simulink library "base_lib"  (R2023a)
settings: Solver=VariableStepAuto  StartTime=0.0  StopTime=10.0  RelTol=1e-3
(part 3 of 4)

== matlab function base_lib/F0010_gasFlow/F0010_mixtureProperties.m ==
  data: p input; x output; cp_m output; cv_m output; R_m output; par parameter
function [x, cp_m, cv_m, R_m] = F0010_mixtureProperties(p, par)
% Parameters
cp_j = par.cp_j; % [J/kgK]  - Specific heats
M_j  = par.M_j;  % [kg/mol] - Molar masses
R_j  = par.R_j;  % [J/kgK]  - Specific gas constant

% Mole fractions
p_tot = sum(p);
x     = p ./ p_tot;

% Average molar mass
M_avg = sum(x .* M_j);

% Mole fraction to mass fraction
w = x .* M_j ./ M_avg;

% Mixture gas constant
R_m = sum(w .* R_j);

% Mixture specific heats
cp_m = sum(w .* cp_j);
cv_m = cp_m - R_m;

end

== matlab function base_lib/F0001_panasonicCell/F0001_ocvSOC.m ==
  data: SOC input; U output
% A Generalized SOC-OCV Model for Lithium-Ion
% Batteries and the SOC Estimation for LNMCO Battery
% Zhang et al, Energies
% doi:10.3390/en9110900

% Fit to OCV-data from
% Li-Ion Battery Model Performance for Automotive Drive
% Cycles with Current Pulse and EIS Parameterization
% Kolmeyer et al, 
% 978-1-5090-3953-1/$31.00 ©2017 IEEE

function U = F0001_ocvSOC(SOC)
% inputs x [-] - state of charge

% parameters
a =  2.0966;
b = -0.0055;
c = -0.2433;
d =  2.3054;
m =  3.0965;
n =  0.6010;

% OCV
x = SOC;
U = a + b * (-log(x)).^m + c .* x + d.*exp( n.*(x-1));
end

== matlab function base_lib/F0010_gasFlow/F0010_multicomponentFlow.m ==
  data: p_us input; W_split output; W_tot input; par parameter
function W_split = F0010_multicomponentFlow(p_us, W_tot, par)
% Parameters
cp_j = par.cp_j; % [J/kgK]  - Specific heats
M_j  = par.M_j;  % [kg/mol] - Molar masses
R_j  = par.R_j;  % [J/kgK]  - Specific gas constant

% Mole fractions
p_tot = sum(p_us);
x     = p_us ./ p_tot;

% Average molar mass
M_avg = sum(x .* M_j);

% Mole fraction to mass fraction
w = x .* M_j ./ M_avg;

% outlet species convective mass flow
W_split = W_tot .* w;

end

== matlab function base_lib/F0010_gasFlow/F0010_pressureSupply.m ==
  data: p_tot input; p_out output; x_H2_dry input; x_O2_dry input; RH input; p_sat input; par parameter
function p_out = F0010_pressureSupply(p_tot, x_H2_dry, x_O2_dry, RH, p_sat, par)

% mole fraction of vapor
x_H2O = RH .* p_sat ./ p_tot;

% mole fraction hydrogen
x_H2 = (1-x_H2O).*x_H2_dry;

% mole fraction hydrogen
x_O2 = (1-x_H2O).*x_O2_dry;

% mole fraction nitrogen
x_N2 = 1 - x_H2 - x_O2 - x_H2O;




% partial pressures
p_out = [x_H2; x_O2; x_H2O; x_N2] .* p_tot;

end

== matlab function base_lib/F0010_gasFlow/F0010_pressureSupply2.m ==
  data: p_tot input; p_H2 output; x_H2_dry input; x_O2_dry input; RH input; p_sat input; p_O2 output; p_H2O output; p_N2 output; par parameter
function [p_H2, p_O2, p_H2O, p_N2] = F0010_pressureSupply2(p_tot, x_H2_dry, x_O2_dry, RH, p_sat, par)

% mole fraction of vapor
x_H2O = RH .* p_sat ./ p_tot;

% mole fraction hydrogen
x_H2 = (1-x_H2O).*x_H2_dry;

% mole fraction hydrogen
x_O2 = (1-x_H2O).*x_O2_dry;

% mole fraction nitrogen
x_N2 = 1 - x_H2 - x_O2 - x_H2O;

% output
p_H2  = x_H2  .* p_tot;
p_O2  = x_O2  .* p_tot;
p_H2O = x_H2O .* p_tot;
p_N2  = x_N2  .* p_tot;

end

== matlab function base_lib/F0010_gasFlow/F0010_pressureToMass.m ==
  data: p input; m output; T input; par parameter
function m = F0010_pressureToMass(p, T, par)
% parameters
Rj     = par.R_j;
V      = par.V;

% mass
m = p .* V ./ (Rj .* T);
end

== matlab function base_lib/F0010_gasFlow/F0010_throttleArea.m ==
  data: alpha input; A_t output; par parameter
function A_t = F0010_throttleArea(alpha, par)
% model parameters
a0 = par.a0;
a1 = par.a1;
a2 = par.a2;

% effective area
A_t = a0 + a1.*alpha + a2 .* alpha.^2;
end

== matlab function base_lib/F0011_ellipseCompressor/F0011_A.m ==
  data: N_corr_n input; A output; par parameter
function A = F0011_A(N_corr_n, par)
% parameters
u1 = N_corr_n;
u2 = par.C_a(1);
u3 = par.C_a(2);
u4 = par.C_a(3);
u5 = par.Delta_h_max;
u6 = par.Wc_max_map;

% output
A = -( u5./u6 ).*( u2.*u1 ./( (1 + u3.*u1.^2).^u4 ));
end

== matlab function base_lib/F0011_ellipseCompressor/F0011_B.m ==
  data: N_corr_n input; B output; par parameter
function B = F0011_B(N_corr_n, par)
% parameters
u1 = N_corr_n;
u2 = par.C_b(1);
u3 = par.C_b(2);
u4 = par.Delta_h_max;

% output
B = u4 .* ( u2 .* u1.^2 + u3 .* u1.^3 );
end

== matlab function base_lib/F0011_ellipseCompressor/F0011_CUR.m ==
  data: N_corr_n input; CUR output; par parameter
function CUR = F0011_CUR(N_corr_n, par)
% parameters
a1     = par.C_cur(1);
a2     = par.C_cur(2);
a3     = par.C_cur(3);

% Speed ratio
N = N_corr_n;

% output
CUR = a1 + a2.*N.^a3;
end

== matlab function base_lib/F0003_pukrushpan2004/F0003_diffusiveFlow.m ==
  data: lambda_an input; W output; lambda_m input; lambda_ca input; T input; par parameter
function W = F0003_diffusiveFlow(lambda_an, lambda_m, lambda_ca, T, par)

% parameters
A   = par.A_fc; % [cm2] - cell area
t_m = par.t_m;  % [cm]  - membrane thickness

% constants
F     = 96485;  % [C/mol]   - Faradays constant
R     = 8.314;  % [J/(molK] - gas constant 
M_H2O = 0.018;  % [kg/mol]  - water molecular mass

rho_mb_dry = 0.002; % [kg/cm^3] - membrane dry density;
M_mb_dry   = 1.1;   % [kg/mol]  - membrane dry equivalent weight 

% membrane diffusivity
D                  = 1e-6;
D(lambda_m >= 2)   = 1e-6 * (1 + 2*(lambda_m-2));
D(lambda_m >= 3)   = 1e-6 * (3 - 1.67*(lambda_m-3));
D(lambda_m >= 4.5) = 1.25e-6;
D_w                = 12 * D.*exp(2416*(1/303 - 1/T));

% Water concentrations on each side
c_an = rho_mb_dry ./ M_mb_dry .* lambda_an; % [mol/cm3] - water concentration at anode
c_ca = rho_mb_dry ./ M_mb_dry .* lambda_ca; % [mol/cm3] - water concentration at cathode

% Diffusive flow
W = M_H2O .* A .* D_w .* (c_an - c_ca)/t_m;

end

== matlab function base_lib/F0011_ellipseCompressor/F0011_K_loss.m ==
  data: W_corr input; K_loss output; N_corr input; par parameter
function K_loss = F0011_K_loss(W_corr, N_corr, par)
% parameters
rho1   = par.rho1;
D      = par.D_2;
C_loss = par.C_loss;

% output
K_loss = 1 + C_loss .* ( rho1.*D.^3 .* pi/60 ) .* (N_corr./W_corr);
end

== matlab function base_lib/F0011_ellipseCompressor/F0011_PI_ZSL.m ==
  data: N_corr_n input; PI_ZSL output; par parameter
function PI_ZSL = F0011_PI_ZSL(N_corr_n, par)
% parameters
PI_max = par.PI_max_map;
a1     = par.C_PIzs(1);
a2     = par.C_PIzs(2);

% Speed ratio
N = N_corr_n;

% output
PI_ZSL  = 1 + (PI_max - 1) .* ( a1.*N.^a2 );
end

== matlab function base_lib/F0011_ellipseCompressor/F0011_P_c.m ==
  data: W_c input; P_c output; T_us input; T_ds input; par parameter
function P_c = F0011_P_c(W_c, T_us, T_ds, par)
% parameters
cp  = par.Cp_air;

% compressor work
P_c = cp .* W_c .* (T_ds - T_us);
end

== matlab function base_lib/F0011_ellipseCompressor/F0011_Pi_ch.m ==
  data: N_corr_n input; Pi_ch output; par parameter
function Pi_ch = F0011_Pi_ch(N_corr_n, par)
% parameters
PI_max = par.PI_max_map;
a1     = par.C_PIch(1);
a2     = par.C_PIch(2);
a3     = par.C_PIch(3);

% Speed ratio
N = N_corr_n;

% output
Pi_ch  = PI_max .* ( a1 + a2.*N.^a3 );
end

== matlab function base_lib/F0011_ellipseCompressor/F0011_T_ds.m ==
  data: Pi_c input; T_ds output; T_us input; eta_c input; par parameter
function T_ds = F0011_T_ds(Pi_c, T_us, eta_c, par)
% model constants
g = par.gamma_air;

% compressor out temperature (adiabatic)
T_ds = T_us + T_us ./ eta_c .* ( Pi_c.^((g-1)/g)  - 1  );
end

== matlab function base_lib/F0011_ellipseCompressor/F0011_W_ZSL.m ==
  data: N_corr_n input; W_ZSL output; par parameter
function W_ZSL = F0011_W_ZSL(N_corr_n, par)
% parameters
Wc_max = par.Wc_max_map;
a1     = par.C_Wzs(1);
a2     = par.C_Wzs(2);

% Speed ratio
N = N_corr_n;

% output
W_ZSL = Wc_max .* a1 .* N.^a2;
end

== matlab function base_lib/F0011_ellipseCompressor/F0011_W_ch_atan.m ==
  data: N_corr_n input; W_ch_atan output; par parameter
function W_ch_atan = F0011_W_ch_atan(N_corr_n, par)
% parameters
Wc_max = par.Wc_max_map;
a1     = par.C_Wch(1);
a2     = par.C_Wch(2);
a3     = par.C_Wch(3);
a4     = par.C_Wch(4);

% Speed ratio
N = N_corr_n;

% output
W_ch_atan = Wc_max .* (a1 + a2 .* atan( a3.*N - a4));
end

== matlab function base_lib/F0011_ellipseCompressor/F0011_dTq.m ==
  data: Tq_em input; dw_c output; Tq_c input; w_c input; par parameter
function dw_c = F0011_dTq(Tq_em, Tq_c, w_c, par)
% parameters
J_c = par.J_c;
c   = par.c_fric;

% shaft friction
Mf = c .* w_c;

% turbo shaft dynamics
% Model 8.3
dw_c = 1/J_c .* ( Tq_em - Tq_c - Mf);

end

== matlab function base_lib/F0011_ellipseCompressor/F0011_dh_act.m ==
  data: W_c_corr input; dh_act output; K_loss input; B input; A input
function dh_act = F0011_dh_act(W_c_corr, K_loss, B, A)
% inputs
u1 = W_c_corr;
u2 = K_loss;
u3 = B;
u4 = A;

% actual enthalpy change
dh_act = u2 .* ( u3 + u4 .* u1 );

end

== matlab function base_lib/F0011_ellipseCompressor/F0011_dh_is.m ==
  data: Pi_c input; dh_is output; par parameter
function dh_is = F0011_dh_is(Pi_c, par)
% inputs
u1 = Pi_c;

% parameters
cp_air = par.Cp_air;
T_ref  = par.T_ref;
g      = par.gamma_air;

% isentropic enthalpy change
dh_is = cp_air .* T_ref .* ( u1.^((g - 1)./g) - 1 );
end

== matlab function base_lib/F0011_ellipseCompressor/F0011_ellipseModel.m ==
  data: Pi_c input; W_corr output; Pi_ch input; PI_ZSL input; CUR input; W_ZSL input; W_ch input; par parameter
function W_corr = F0011_ellipseModel(Pi_c, Pi_ch, PI_ZSL, CUR, W_ZSL, W_ch, par)
% inputs
u1 = min(Pi_c, PI_ZSL);
u2 = Pi_ch;
u3 = PI_ZSL;
u4 = CUR;
u5 = W_ZSL;
u6 = W_ch;


% inputs
u1 = min(Pi_c, PI_ZSL);
u2 = Pi_ch;
u3 = PI_ZSL;
u4 = CUR;
u5 = W_ZSL;
u6 = W_ch;

% Surge / Regular / Choke
if (Pi_c >  PI_ZSL)
    W_corr = W_ZSL - (Pi_c - PI_ZSL)./par.alpha_kPiW0;
elseif (Pi_c < Pi_ch)
    W_corr = W_ch;
else
    W_corr = u5 + (u6-u5).*( (1 - ( (u1-u2)./(u3-u2) ).^u4).^(1./u4) );
end

== matlab function base_lib/F0011_ellipseCompressor/F0011_ellipseModelPressure.m ==
  data: W_corr input; Pi_c output; Pi_ch input; PI_ZSL input; CUR input; W_ZSL input; W_ch input; par parameter
function Pi_c = F0011_ellipseModelPressure(W_corr, Pi_ch, PI_ZSL, CUR, W_ZSL, W_ch, par)

% inputs
W_corr = min(W_corr, W_ch);
W_corr = max(W_corr, W_ZSL);

% Surge / Regular / Choke
if (W_corr <  W_ZSL)
    Pi_c = PI_ZSL;
elseif (W_corr > W_ch)
    Pi_c = Pi_ch;
else
    Pi_c   = Pi_ch + ...
    (PI_ZSL - Pi_ch) .* ... 
    (1 - ((W_corr - W_ZSL)./(W_ch - W_ZSL)).^CUR ).^(1./CUR);
end

== matlab function base_lib/F0003_pukrushpan2004/F0003_dragFlow.m ==
  data: I input; W output; lambda input
function W = F0003_dragFlow(I, lambda)

% parameters
F          = 96485;  % [C/mol]   - Faradays constant
M_H2O      = 0.018;  % [kg/mol]  - water molecular mass

% electro-osmotic drag coefficient
n_d = 0.0029 .* lambda.^2 + 0.05 .* lambda;

% Drag flow
W =  M_H2O .* n_d .* I / F;
end

== matlab function base_lib/F0011_ellipseCompressor/F0011_flowCorrection.m ==
  data: W_c input; W_corr output; p1 input; T1 input; par parameter
function W_corr = F0011_flowCorrection(W_c, p1, T1,  par)

% corrected flow
W_corr = W_c .* sqrt( T1./par.T_ref) ./ (p1./par.p_ref);

end

== matlab function base_lib/F0011_ellipseCompressor/F0011_linearSurgeFlow.m ==
  data: W_ZSL input; W_corr_surge output; Pi_ZSL input; Pi_c input; par parameter
function W_corr_surge = F0011_linearSurgeFlow(W_ZSL, Pi_ZSL, Pi_c, par)
% Surge flow
W_corr_surge = W_ZSL - (Pi_c - Pi_ZSL)./par.alpha_kPiW0;

% Saturation
W_corr_surge(W_corr_surge < 1e-4) = 1e-4;
end

== matlab function base_lib/F0014_titanXradiator/F0014_condenserPressureDrop.m ==
  data: T input; dp output; p input; W input; par parameter
function dp = F0014_condenserPressureDrop(T, p, W, par)

% parameters
StS  = par.StS;
HtH  = par.HtH;
R    = par.R_air;
c_dp = par.c_dp; 

% Area
A = StS .* HtH;

% Velocity
v = W .* R .* T ./ (p.*A);

% pressure drop
dp = c_dp(1) .* v.^2 + c_dp(2) .* v;

== matlab function base_lib/F0014_titanXradiator/F0014_coreFlowDelay.m ==
  data: W input; t output; rho input; par parameter
function t = F0014_coreFlowDelay(W, rho, par)

% parameters
HtH = par.HtH;
StS = par.StS;
CdT = par.CdT;

% approximate core inner flow area
A = 0.15 .* CdT .* StS;

% flow velocity
v = max(W ./ ( rho .* A), 0.01);

% time delay
t = min(HtH ./ v, 20);

== matlab function base_lib/F0014_titanXradiator/F0014_epsCrossFlowUnmixed.m ==
  data: NTU input; e output; C input
function e = F0014_epsCrossFlowUnmixed(NTU, C)
N = NTU;
% N = max(N, 0);
n = N.^(-0.22);

% tanhyp switch for C approaching zero
y = (tanh(C*1e2 - pi) + 1 )./2;

% Holman, Table 10.3, Cross flow, both fluids unmixed:
e1  = 1 - exp( ( exp( -N.*C.*n ) - 1 )./(C.*n) );

% C = 0
e0 = 1 - exp(-N);

% output
e = y.*e1 + (1-y).*e0;

== matlab function base_lib/F0014_titanXradiator/F0014_fanAffinityLaw.m ==
  data: n1 input; q1 output; q2 input; dp1 output; P1 output; par parameter
function [q1, dp1, P1] = F0014_fanAffinityLaw(n1, q2, par)
% Source:
% https://www.engineeringtoolbox.com/fan-affinity-laws-d_196.html

% parameters
dp2 = par.dp2;
P2  = par.P2;
n2  = par.n2;
d1  = par.d1;
d2  = par.d2;

% Affinity laws
q1  = q2  .* (n1./n2)    .* (d1./d2).^3;
dp1 = dp2 .* (n1./n2).^2 .* (d1./d2).^2;
P1  = P2  .* (n1./n2).^3 .* (d1./d2).^5;

== matlab function base_lib/F0014_titanXradiator/F0014_fanCurve.m ==
  data: q input; dp output; dp0_n input; par parameter
function dp = F0014_fanCurve(q, dp0_n, par)

% parameters
dpr = par.dpr;
dp0 = par.dp0;
q0  = par.q0;

% pressure drop/increase
temp = (q ./ q0).^2;
dp   = max(dpr .* temp, dp0_n - dp0 .* temp);

== matlab function base_lib/F0014_titanXradiator/F0014_heatCapacityRates.m ==
  data: W_air input; C_min output; W_cl input; cp_cl input; C_max output; C_air output; C_cl output; par parameter
function [C_min, C_max, C_air, C_cl] = F0014_heatCapacityRates(W_air, W_cl, cp_cl, par)

% parameters
cp_air = par.cp_air;
% cp_clt = par.cp_clt;

% heat capacity rates
C_air = W_air.*cp_air;
C_cl = W_cl.*cp_cl;

% max/min rates
C_min = min(C_air, C_cl);
C_max = max(C_air, C_cl);

== matlab function base_lib/F0003_pukrushpan2004/F0003_outputVoltage.m ==
  data: I input; V output; p_an input; p_ca input; p_sat input; lambda_m input; T input; Q_gen output; par parameter
function [V, Q_gen] = F0003_outputVoltage(I, p_an, p_ca, p_sat, lambda_m, T, par)
% ref: Control-Oriented Modeling and Analysis for Automotive Fuel Cell Systems
% authors: Jay T. Pukrushpan, Huei Peng, Anna G. Stefanopoulou
% J. Dyn. Sys., Meas., Control. Mar 2004
% https://doi.org/10.1115/1.1648308

% specify output sizes
Q_gen = 0;
V     = 0;

% parameters
A = par.A_fc; % [cm2]       - cell area
j = I ./ A;

% partial pressures
p_H2     = p_an(1); % [Pa] - hydrogen partial pressure
% p_H2O_an = p_an(2); % [Pa] - water --
% p_N2_an  = p_an(3); % [Pa] - nitrogen --
p_O2     = p_ca(2); % [Pa] - oxygen --
p_H2O_ca = p_ca(3); % [Pa] - water --
p_N2_ca  = p_ca(4); % [Pa] - nitrogen --

% parameters
c1 = 10;

% constants
R     = 8.314;     % [J/(K mol)] - Gas constant
F     = 96485;     % [C/mol]     - Faradays constant
n     = 2;         % [-]         - moles of electrons transfered per mole hydrogen reacted
E0    = 1.229;     % [V]         - standard potential
P_atm = 1.01325e5; % [Pa]        - atm. pressure
p0    = 1e5;       % [Pa]        - std. pressure
dh    = 285.8e3;   % [J/mol]     - heat of formation (liquid)
% dh    = 241.8e3;   % [J/mol]     - heat of formation (vapor)

% total pressures
% P_an = p_H2 + p_H2O_an + p_N2_an;
P_ca = p_O2 + p_H2O_ca + p_N2_ca;

% reversible voltage
% E = E0 - 8.5e-4 .* (T-298.15) + R*T/(n*F) * log(p_H2./p0 .* sqrt( max(p_O2./p0,0) ));
E = E0 - 8.5e-4 .* (T-298.15) + R*T/(n*F) * log(p_H2./p0 .* sqrt( p_O2./p0 ));


% activation overvoltage
v0 = 0.279 - 8.5e-4 .* (T - 298.15) + 4.3085e-5 .* T .* (log((P_ca/P_atm - p_sat./P_atm)/1.01325) + 1/2 * log(0.1173*(P_ca/P_atm - p_sat./P_atm)/1.01325));
va = (-1.618e-5 * T + 1.618e-2) .* ( p_O2./P_atm./0.1173 + p_sat./P_atm ).^2 + (1.8e-4 * T - 0.166).*(p_O2./ P_atm/0.1173 + p_sat./P_atm) + (-5.8e-4 * T + 0.5736);
V_act = v0 + va.*(1 - exp(-c1.*j));

% ohmic overvoltage
b11     = 0.005139;
b12     = 0.00326;
b2      = 350;
t_m     = 0.01275;
sigma_m = (b11 .* max(lambda_m,1) - b12) .* exp( b2 .*( 1./303 - 1./T ) );
R_ohm   = t_m ./ sigma_m;
V_ohm   = j .* R_ohm;

% concentration overvoltage
temp         = (p_O2./P_atm./0.1173 + p_sat./P_atm);
c2           = (8.66e-5 .* T - 0.068) .* temp + ( -1.60e-4 * T + 0.54);
% c2(temp < 2) = (7.16e-4 .* T - 0.622) .* temp + ( -1.45e-3 * T + 1.68);
c3           = 2;
j_max        = 2.2;
V_con        = j .* (c2 .* j/j_max).^c3;

% Output voltage
% V = E  - V_act - V_ohm - V_con;
V = E  - V_act - V_ohm - V_con;

% Heat generation
P_elec = j.*A .* V;              % [W] - electric power
P_tot  = j .*A ./ (2*F) .* dh;   % [W] - total power
Q_gen  = P_tot - P_elec;         % [W] - heat generation

== matlab function base_lib/F0014_titanXradiator/F0014_intakePressureIncrease.m ==
  data: T input; dp output; p input; v input; par parameter
function dp = F0014_intakePressureIncrease(T, p, v, par)

% parameters
zeta = par.zeta;
R    = par.R_air;

% density
rho = p ./ (R.*T);

% pressure drop
dp = 1/2 .* zeta .* rho .* v.^2;

== matlab function base_lib/F0014_titanXradiator/F0014_radiatorAirPressureDrop.m ==
  data: v input; dp output; par parameter
function dp = F0014_radiatorAirPressureDrop(v, par)
% parameters
CdT   = par.CdT;
c_dp  = par.c_dp_air;
rho   = par.rho_air;

% pressure drop
dp = CdT .* rho .* ( c_dp(1) .* v.^2 + c_dp(2) .* v );

== matlab function base_lib/F0014_titanXradiator/F0014_radiatorCltPressureDrop.m ==
  data: v input; dp output; rho input; par parameter
function dp = F0014_radiatorCltPressureDrop(v, rho, par)
% parameters
HtH   = par.HtH;
c_dp  = par.c_dp_clt;

% pressure drop
dp = HtH .* rho .* ( c_dp(1) .* v.^2 + c_dp(2) .* v );

== matlab function base_lib/F0014_titanXradiator/F0014_restrictionPressureDrop.m ==
  data: T input; dp output; p input; W input; par parameter
function dp = F0014_restrictionPressureDrop(T,p,W,par)

% parameters
zeta = par.zeta;
R    = par.R_air;
A    = par.A;

% density
rho = p ./ (R.*T);

% velocity
v = W ./ (rho.*A);

% pressure drop
dp = 1/2 .* zeta .* rho .* v.^2;

== matlab function base_lib/F0014_titanXradiator/F0014_restrictionPressureDrop2.m ==
  data: T input; dp output; p input; W input; par parameter
function dp = F0014_restrictionPressureDrop2(T,p,W,par)

% parameters
zeta = par.zeta;
R    = par.R_air;

% density
rho = p ./ (R.*T);

% pressure drop
dp = zeta .* W.^2 ./ rho;

== matlab function base_lib/F0014_titanXradiator/F0014_tankPressureDrop.m ==
  data: v input; dp output; par parameter
function dp = F0014_tankPressureDrop(v, par)
% parameters
zeta = par.zeta;

% pressure drop
dp = 1/2 .* v .* abs(v) .* zeta;

== matlab function base_lib/F0017_channelCooling/F0017_Nusselt.m ==
  data: Re input; Nu output; Pr input; par parameter
function Nu = F0017_Nusselt(Re, Pr, par)

% parameters
d = par.d;
L = par.L;

% Hausen Nusselt Correlation:
Nu_lam = 3.66 + ...
    (0.0668.*(d./L) .* Re .* Pr) ./ ...
    (1 + 0.04 .*( max( (d./L) .* Re .* Pr , 1e-10) ).^(2/3) );

% Sieder-Tate Correlation:
Nu_turb = 0.027 .* Re.^0.8 .* Pr.^(1/3);

% transition from laminar to turbulent flow
y = (Re-3500) / 2e3;
y = tanh(y*5)/2 + 1/2;

% Nusselt number
Nu = (1-y) .* Nu_lam + y.*Nu_turb;

== matlab function base_lib/F0017_channelCooling/F0017_Prandtl.m ==
  data: cp input; Pr output; mu input; lam input; par parameter
function Pr = F0017_Prandtl(cp, mu, lam, par)

% Prandtl number
Pr = cp .* mu ./ lam;

== matlab function base_lib/F0017_channelCooling/F0017_Reynolds.m ==
  data: v input; Re output; rho input; mu input; par parameter
function Re = F0017_Reynolds(v, rho, mu, par)
% parameters
d   = par.d;

% Pipe reynolds number
Re = rho .* v .* d ./ mu;

== matlab function base_lib/F0017_channelCooling/F0017_enthalpyToTemperature.m ==
  data: H input; T output; cp input; H0 input; T0 input; par parameter
function T = F0017_enthalpyToTemperature(H, cp, H0, T0, par)
    
    % temperature
    T = T0 + 1./cp .* (H - H0);

end

== matlab function base_lib/F0017_channelCooling/F0017_heatTransfer.m ==
  data: T_1 input; Q output; T_w input; Nu input; W input; cp input; lam input; T_2 output; par parameter
function [Q, T_2] = F0017_heatTransfer(T_1, T_w, Nu, W, cp, lam, par)
% Holman example 6-2, Heating of water in Laminar tube flow
% parameters
d    = par.d;
L    = par.L;

% heat transfer coefficient
h = lam .* Nu ./ d;

% factors
c1 =  W .* cp; 
c2 =  h.*pi.*d.*L;

% outlet temperature
T_2p = (c2 .* T_w + (c1 - c2./2) .* T_1 )./(c1 + c2./2);

% check if temperature reaches wall temperature
if T_1 < T_w
    % cooling
    T_2 = min(T_2p, T_w);
else
    % heating
    T_2 = max(T_2p, T_w);
end
   
% heat transfer
Q = W .* cp .* (T_2 - T_1);

== matlab function base_lib/F0017_channelCooling/F0017_heatTransfer2.m ==
  data: T_1 input; Q output; T_w input; Nu input; W input; cp input; lam input; T_2 output; par parameter
function [Q, T_2] = F0017_heatTransfer2(T_1, T_w, Nu, W, cp, lam, par)
% Holman example 6-2, Heating of water in Laminar tube flow
% parameters
d  = par.d;
L  = par.L;

% heat transfer coefficient
h = lam .* Nu ./ d;

% factors
c1 =  W .* cp; 
c2 =  h.*pi.*d.*L;

% outlet temperature
T_2p = (c2 .* T_w + (c1 - c2./2) .* T_1 )./(c1 + c2./2);

% variable for cooling or heating mode
tmp = (T_1 - T_w)/1e1;            % Cooling when negative
y   = (tanh(tmp) + 1)/2;

% outlet temperature
T_2_cool = min(T_2p, T_w);
T_2_heat = max(T_2p, T_w);
T_2      = (1-y) .* T_2_cool + y .* T_2_heat;

% cooling
% T_2 = min(T_2p, T_w)

% heat transfer
Q = W .* cp .* (T_2 - T_1);

== matlab function base_lib/F0017_channelCooling/F0017_incompressibleRestriction.m ==
  data: W input; dp output; dr input; rho input; par parameter
function dp = F0017_incompressibleRestriction(W, dr, rho,  par)

% parameters
C_d = par.C_d;
d   = par.d;

% restriction area
Ar = dr.^2 * pi / 4;

% diameter ratio
beta = dr./d;

% volumetric flow
% Q = W ./ rho;

% pressure drop
% dp = 1/2 .* rho .* (1 - beta.^4) .* (W ./ (C_d .* Ar)).^2;
dp = 1/rho .* (1 - beta.^4) .* (W ./ (C_d .* Ar)).^2;

== matlab function base_lib/F0003_pukrushpan2004/F0003_outputVoltage2.m ==
  data: I input; V output; p_tot input; p_H2 input; p_O2 input; p_sat input; lambda_m input; T input; Q_gen output; par parameter
function [V, Q_gen] = F0003_outputVoltage2(I, p_tot, p_H2, p_O2, p_sat, lambda_m, T, par)
% ref: Control-Oriented Modeling and Analysis for Automotive Fuel Cell Systems
% authors: Jay T. Pukrushpan, Huei Peng, Anna G. Stefanopoulou
% J. Dyn. Sys., Meas., Control. Mar 2004
% https://doi.org/10.1115/1.1648308

% specify output sizes
Q_gen = 0;
V     = 0;

% parameters
A = par.A_fc; % [cm2]       - cell area
j = I ./ A;

% % partial pressures
% p_H2     = p_an(1); % [Pa] - hydrogen partial pressure
% p_O2     = p_ca(2); % [Pa] - oxygen --
% p_H2O_ca = p_ca(3); % [Pa] - water --
% p_N2_ca  = p_ca(4); % [Pa] - nitrogen --

% parameters
c1 = 10;

% constants
R     = 8.314;     % [J/(K mol)] - Gas constant
F     = 96485;     % [C/mol]     - Faradays constant
n     = 2;         % [-]         - moles of electrons transfered per mole hydrogen reacted
E0    = 1.229;     % [V]         - standard potential
P_atm = 1.01325e5; % [Pa]        - atm. pressure
p0    = 1e5;       % [Pa]        - std. pressure
dh    = 285.8e3;   % [J/mol]     - heat of formation (liquid)
% dh    = 241.8e3;   % [J/mol]     - heat of formation (vapor)

% total pressures
% P_an = p_H2 + p_H2O_an + p_N2_an;
P_ca = p_tot;

% reversible voltage
% E = E0 - 8.5e-4 .* (T-298.15) + R*T/(n*F) * log(p_H2./p0 .* sqrt( max(p_O2./p0,0) ));
E = E0 - 8.5e-4 .* (T-298.15) + R*T/(n*F) * log(p_H2./p0 .* sqrt( p_O2./p0 ));


% activation overvoltage
v0 = 0.279 - 8.5e-4 .* (T - 298.15) + 4.3085e-5 .* T .* (log((P_ca/P_atm - p_sat./P_atm)/1.01325) + 1/2 * log(0.1173*(P_ca/P_atm - p_sat./P_atm)/1.01325));
va = (-1.618e-5 * T + 1.618e-2) .* ( p_O2./P_atm./0.1173 + p_sat./P_atm ).^2 + (1.8e-4 * T - 0.166).*(p_O2./ P_atm/0.1173 + p_sat./P_atm) + (-5.8e-4 * T + 0.5736);
V_act = v0 + va.*(1 - exp(-c1.*j));

% ohmic overvoltage
b11     = 0.005139;
b12     = 0.00326;
b2      = 350;
t_m     = 0.01275;
sigma_m = (b11 .* max(lambda_m,1) - b12) .* exp( b2 .*( 1./303 - 1./T ) );
R_ohm   = t_m ./ sigma_m;
V_ohm   = j .* R_ohm;

% concentration overvoltage
temp         = (p_O2./P_atm./0.1173 + p_sat./P_atm);
c2           = (8.66e-5 .* T - 0.068) .* temp + ( -1.60e-4 * T + 0.54);
% c2(temp < 2) = (7.16e-4 .* T - 0.622) .* temp + ( -1.45e-3 * T + 1.68);
c3           = 2;
j_max        = 2.2;
V_con        = j .* (c2 .* j/j_max).^c3;

% Output voltage
% V = E  - V_act - V_ohm - V_con;
V = E  - V_act - V_ohm - V_con;

% Heat generation
P_elec = j.*A .* V;              % [W] - electric power
P_tot  = j .*A ./ (2*F) .* dh;   % [W] - total power
Q_gen  = P_tot - P_elec;         % [W] - heat generation

== matlab function base_lib/F0017_channelCooling/F0017_pressureDrop.m ==
  data: v input; dp output; Re input; rho input; par parameter
function dp = F0017_pressureDrop(v, Re, rho,  par)
% parameters
d   = par.d;
L   = par.L;
e   = par.e;

% Darcy-weisbach friction factor
% laminar
f_lam = 64 ./ (Re + 0.01);

% turbulent and roughness
kd     = e./d;
f_turb = 1./(-1.8 .* log10(6.9 ./ (Re+0.001) + (kd./3.7).^(10/9) )).^2;

% smooth transition between laminar & turbulent
y = (Re-2100) / 500;
y = tanh(y*5)/2 + 1/2;

% combined
f = y .* f_turb + (1-y).* f_lam;

% pressure drop
dp =  L .* f .* rho./2 .* v.^2 ./ d;

== matlab function base_lib/F0017_channelCooling/F0017_restriction.m ==
  data: W input; dp output; rho input; par parameter
function dp = F0017_restriction(W, rho, par)

% Discharge coefficient
C   = par.C;
d   = par.d;

% Area
A = pi .* d.^2 / 4;

% Laminar restriction
dp = 1./rho .* (W ./ (C.*A));

== matlab function base_lib/F0018_ambientProperties/F0018_troposphereModel.m ==
  data: h input; p output; T output; par parameter
function [p,T] = F0018_troposphereModel(h, par)

% parameters
T_0 = par.T_0;
p_0 = par.p_0;

% The nasa troposphere model for pressure.
T = T_0 - 0.00649 .* h;
p = p_0 .* (T./288.078).^5.256;

== matlab function base_lib/F0019_simpleCompressor/F0007_compressorPower.m ==
  data: W_c input; P_c output; T_us input; T_ds input
function P_c = F0007_compressorPower(W_c, T_us, T_ds)

% model constants
g   = 1.4;
R   = 280;
cp  = g*R/(g-1);

% compressor work
P_c = cp .* W_c .* (T_ds - T_us);

end

== matlab function base_lib/F0019_simpleCompressor/F0007_compressorTemperature.m ==
  data: p_us input; T_ds output; p_ds input; T_us input; eta_c input
function T_ds = F0007_compressorTemperature(p_us, p_ds, T_us, eta_c)

% model constants
g = 1.4;

% pressure ratio
PiC = p_ds./p_us;

% compressor out temperature (adiabatic)
T_ds = T_us + T_us ./ eta_c .* ( PiC.^((g-1)/g)  - 1  );

end

== matlab function base_lib/F0020_dcdcConverter/F0020_dcdcConverter.m ==
  data: U_bus input; eta output; U_s input; I input; I_bus output; P_bus output; Q_gen output; par parameter
function [eta, I_bus, P_bus, Q_gen] = F0020_dcdcConverter(U_bus, U_s, I, par)
% Function for the DC-DC converter connected to a DC-bus. The system
% connected to the converter can be either a consumer or a producer.
% Negative current, I, means that the connected device is a consumer from
% the DC-bus and a positive current means that the connected device is a
% producer to the DC-bus.


% Output:
% - eta: Voltage change efficiency
% - I_bus: Current to and from the DC Bus.
% - P_bus: Power to and from the DC Bus
% - P_loss: Converting loss, always positive.
% Inputs:
% - U_bus: DC Bus Voltage
% - U_s: System voltage connected to converter
% - I: Current to DC Bus (negative current is a consumer, positive a producer.)
% - eta_down: Buck Efficiency
% - eta_up: Boost Efficiency


% parameters
eta_down = par.eta_down;
eta_up   = par.eta_up;


producer = false;
U_out = 0;
U_in  = 0;

% producer/consumer mode:
if( I < 0 ) 
    % ... consumer from bus
    U_out = U_s;
    U_in  = U_bus;
else
    % ... producer to bus
    producer = true;
    U_out    = U_bus;
    U_in     = U_s;
end

% buck/boost mode:
if( U_out < U_in )
    % Buck conversion
    eta = eta_down;
else 
    % Boost conversion
    eta = eta_up;
end


P_s = U_s*I;

if( producer )
    P_bus = P_s*eta;
    I_bus = P_bus/U_bus;
else
    P_bus = P_s/eta;
    I_bus = P_bus/U_bus;
end

% heat generation
% P_bus < P_s < 0 for consumer current.
Q_gen = P_s-P_bus; 

end

== matlab function base_lib/F0021_R1234yf/F0021_Tsat.m ==
  data: p input; Tsat output
function Tsat = F0021_Tsat(p)

% critical properties
Tc   =     367.85; % [K]
pc   = 	3382200.0; % [Pa]
rhoc =     4170.0; % [mol/m3]

p = max(p,0);
p = min(p, pc);

% coefficients
x = [ 0.011785783765939;
  -0.000711388291699;
  -0.000000004534501;
   0.000005602194397;
   0.000000550569193 ];

% calculate saturated temperature
pr   = p ./ pc;
A    = [ones(size(p)), log(pr), log(pr).^2, log(pr).^3, log(pr).^4];
Tsat = exp( ( A * x ).^(-0.4) );

end

== matlab function base_lib/F0021_R1234yf/F0021_a.m ==
  data: T input; a output; rho input
function a = F0021_a(T,rho)
%R1234yf_a
%    A = R1234yf_a(T,RHO)

%    This function was generated by the Symbolic Math Toolbox version 9.3.
%    16-Oct-2023 15:47:49

t2 = rho.^2;
t3 = rho.^3;
t4 = 1.0./T;
t5 = rho./4.17e+3;
t6 = -t5;
t8 = t4.*3.6785e+2;
t9 = t2./1.73889e+7;
t7 = exp(t6);
t10 = -t9;
t11 = t8.^(7.0./2.0);
t12 = exp(t10);
et1 = t4.*2.95847224925e+3+log(-exp(t4.*-7.18e+2)+1.0).*7.549+log(-exp(t4.*-8.77e+2)+1.0).*1.537+log(-exp(t4.*-1.755e+3)+1.0).*7.455+log(-exp(t4.*-4.465e+3)+1.0).*(2.03e+2./1.0e+2)+log(t5)+log(t8).*(6.18e+2./1.25e+2)+rho.*t8.^(8.0./2.5e+1).*3.709731414868106e-4;
et2 = rho.*t8.^(9.29e+2./1.0e+3).*(-5.64805035971223e-4)+t2.^2.*t4.*5.587038487243495e-14+t3.*t8.^(1.9e+1./5.0e+1).*2.424466237613225e-12;
et3 = t2.*t8.^(4.7e+1./5.0e+1).*(-2.776388960773827e-8)-rho.*t8.^(5.7e+1./2.5e+1).*t12.*2.901693045563549e-4-t3.*t8.^(4.4e+1./2.5e+1).*t12.*8.518739586251397e-12;
et4 = t2.*t8.^(6.1e+1./2.5e+1).*t12.*(-4.007473158164116e-8)+t2.*t7.*t8.^(9.7e+1./1.0e+2).*3.913566700596357e-8+t2.*t11.*exp((t8-6.0./5.0).^2.*-1.08e+2-(t5-4.1e+1./2.5e+1).^2.*(8.1e+1./5.0)).*1.971683660266032e-11;
et5 = t3.*t4.*exp((t8-3.2e+1./2.5e+1).^2.*-8.0e+1-(t5-3.59e+2./5.0e+2).^2.*(1.46e+2./2.5e+1)).*(-5.821977769301905e-9)-t3.*t11.*exp((t8-2.3e+1./5.0e+1).^2.*(-8.9e+1./1.0e+2)-(t5-6.77e+2./1.0e+3).^2.*(2.11e+2./2.0e+2)).*2.723951646267135e-12;
et6 = rho.^7.*t7.*t8.^(2.1e+1./2.0e+1).*(-1.229509534838242e-27)+rho.*t8.^(7.0./5.0).*exp((t5-8.9e+1./1.25e+2).^2.*(-5.1e+1./5.0e+1)-(t8-1.13e+2./1.0e+2).^2.*(7.1e+1./5.0e+1)).*3.333251798561151e-4;
et7 = rho.*t4.^3.*exp((t8-6.7e+1./1.0e+2).^2.*(-2.31e+2./1.0e+2)-(t5-9.1e+1./1.0e+2).^2.*(1.67e+2./1.25e+2)).*(-5.702218194789895e+3)-1.2837928e+1;
a = T.*(et1+et2+et3+et4+et5+et6+et7).*8.314472;
end

== matlab function base_lib/F0021_R1234yf/F0021_cp.m ==
  data: T input; cp output; rho input
function cp = F0021_cp(T,rho)
%R1234yf_cp
%    CP = R1234yf_cp(T,RHO)

%    This function was generated by the Symbolic Math Toolbox version 9.3.
%    16-Oct-2023 15:47:52

t2 = rho.^2;
t3 = rho.^3;
t5 = rho.^5;
t7 = rho.^7;
t8 = 1.0./T;
t11 = rho./4.17e+3;
t16 = rho.*7.769784172661871e-3;
t24 = rho.*4.892086330935252e-4;
t29 = rho.*2.800959232613909e-3;
t31 = rho.*6.407673860911271e-4;
t32 = rho.*5.059952038369305e-4;
t4 = t2.^2;
t6 = t2.^3;
t9 = t8.^2;
t10 = t8.^3;
t12 = t8.*7.18e+2;
t13 = t8.*8.77e+2;
t14 = t8.*1.755e+3;
t15 = t8.*4.465e+3;
t17 = -t11;
t22 = t8.*5.8856e+4;
t30 = t8.*3.6785e+2;
t33 = t8.*7.94556e+4;
t34 = t2./1.73889e+7;
t39 = t8.*1.044694e+3;
t40 = t11-4.1e+1./2.5e+1;
t48 = t8.*6.54773e+2;
t49 = t8.*1.699467e+3;
t50 = t11-9.1e+1./1.0e+2;
t51 = t11-8.9e+1./1.25e+2;
t52 = t11-3.59e+2./5.0e+2;
t67 = t11-6.77e+2./1.0e+3;
t68 = t16-5.3136e+1;
t77 = t24-1.45248;
t86 = t29-8.38624;
t91 = t31-2.43152;
t99 = t32-1.42847;
t122 = t3.*t8.*9.319180196722149e-10;
t18 = -t12;
t19 = -t13;
t20 = -t14;
t21 = -t15;
t23 = exp(t17);
t41 = -t34;
t42 = t30.^(3.0./2.0);
t43 = t30.^(2.0./5.0);
t44 = t30.^(5.0./2.0);
t45 = t30.^(7.0./2.0);
t46 = t30.^(7.0./5.0);
t53 = t30-6.0./5.0;
t54 = t30.^(1.0./2.0e+1);
t55 = t40.^2;
t56 = t30.^(8.0./2.5e+1);
t58 = t30.^(1.9e+1./2.5e+1);
t60 = t30.^(3.6e+1./2.5e+1);
t61 = t30.^(1.9e+1./5.0e+1);
t62 = t30.^(4.4e+1./2.5e+1);
t64 = t30.^(6.1e+1./2.5e+1);
t65 = t30.^(4.7e+1./5.0e+1);
t66 = t22-2.048e+2;
t69 = t30-3.2e+1./2.5e+1;
t70 = t30-2.3e+1./5.0e+1;
t71 = 1.0./t30.^(3.0./1.0e+2);
t72 = t50.^2;
t73 = t51.^2;
t74 = t52.^2;
t76 = t30.^(9.7e+1./1.0e+2);
t78 = t30-6.7e+1./1.0e+2;
t79 = t30-1.13e+2./1.0e+2;
t80 = t33-2.592e+2;
t81 = t67.^2;
t84 = t30.^(9.29e+2./1.0e+3);
t96 = t39-3.2092;
t102 = t48-8.188e-1;
t105 = t49-3.0954;
t25 = exp(t18);
t26 = exp(t19);
t27 = exp(t20);
t28 = exp(t21);
t47 = exp(t41);
t57 = t54.^21;
t59 = t56.^4;
t63 = t58.^3;
t75 = t53.^2;
t82 = t69.^2;
t83 = t70.^2;
t87 = t78.^2;
t88 = t79.^2;
t89 = t55.*(8.1e+1./5.0);
t94 = t73.*(5.1e+1./5.0e+1);
t98 = t74.*(1.46e+2./2.5e+1);
t100 = t72.*(1.67e+2./1.25e+2);
t106 = t81.*(2.11e+2./2.0e+2);
t114 = t56.*1.546958;
t118 = t84.*2.355237;
t119 = rho.*t65.*2.315508393285372e-4;
t129 = t2.*t61.*3.033007263254145e-8;
t132 = rho.*t23.*t76.*3.263914628297362e-4;
t135 = t2.*t23.*t76.*3.913566700596357e-8;
t35 = t25-1.0;
t36 = t26-1.0;
t37 = t27-1.0;
t38 = t28-1.0;
t85 = t75.*1.08e+2;
t92 = -t89;
t93 = t82.*8.0e+1;
t97 = -t94;
t101 = -t98;
t103 = -t100;
t104 = t83.*(8.9e+1./1.0e+2);
t108 = t88.*(7.1e+1./5.0e+1);
t109 = -t106;
t111 = t87.*(2.31e+2./1.0e+2);
t120 = -t118;
t121 = -t119;
t130 = t47.*t63.*1.210006;
t133 = rho.*t47.*t64.*3.342232613908873e-4;
t136 = t2.*t47.*t63.*1.391699302428561e-7;
t137 = -t135;
t138 = t2.*t47.*t62.*1.06569432224005e-7;
t140 = t3.*t47.*t64.*1.922049476337705e-11;
t141 = t4.*t47.*t62.*4.085726420264459e-15;
t142 = t6.*t23.*t57.*3.588938332192827e-23;
t144 = t7.*t23.*t57.*1.229509534838242e-27;
t90 = -t85;
t95 = -t93;
t107 = -t104;
t110 = -t108;
t112 = -t111;
t131 = -t130;
t134 = -t133;
t139 = -t138;
t143 = -t142;
t113 = t90+t92;
t116 = t95+t101;
t123 = t97+t110;
t125 = t103+t112;
t126 = t107+t109;
t115 = exp(t113);
t117 = exp(t116);
t124 = exp(t123);
t127 = exp(t125);
t128 = exp(t126);
t145 = t2.*t8.*t117.*7.283294189396684e-5;
t147 = rho.*t45.*t115.*1.644384172661871e-7;
t148 = t46.*t124.*1.389966;
t149 = t10.*t127.*2.377824987227386e+7;
t151 = t2.*t45.*t128.*3.407663509480186e-8;
t153 = t3.*t8.*t86.*t117.*5.821977769301905e-9;
t154 = t2.*t45.*t68.*t115.*1.971683660266032e-11;
t156 = rho.*t46.*t77.*t124.*3.333251798561151e-4;
t158 = rho.*t10.*t91.*t127.*5.702218194789895e+3;
t159 = t3.*t45.*t99.*t128.*2.723951646267135e-12;
t146 = -t145;
t150 = -t149;
t152 = -t151;
t155 = -t154;
t157 = -t156;
t160 = t114+t120+t121+t122+t129+t131+t132+t134+t136+t137+t139+t140+t141+t143+t144+t146+t147+t148+t150+t152+t153+t155+t157+t158+t159;
et1 = 1.0./t35.^2.*exp(t8.*-1.436e+3).*2.876052391546904e+1+1.0./t36.^2.*exp(t8.*-1.754e+3).*8.736380352244283+1.0./t37.^2.*exp(t8.*-3.51e+3).*1.696916093943165e+2+1.0./t38.^2.*exp(t8.*-8.93e+3).*2.990869359808914e+2+rho.*t71.^56.*8.072375558752998e-5;
et2 = rho.*1.0./t30.^1.071.*(-3.72539753676259e-5)-(t25.*2.876052391546904e+1)./t35-(t26.*8.736380352244283)./t36-(t27.*1.696916093943165e+2)./t37-(t28.*2.990869359808914e+2)./t38;
et3 = t3.*t71.^54.*5.712042455816759e-13-t2.*1.0./t30.^(5.3e+1./5.0e+1).*1.565883373876438e-9+3.653734124219459e-5./t9+rho.*t30.^(7.0./2.5e+1).*t47.*8.468300984172661e-4;
et4 = rho.*1.0./t54.^12.*t124.*(-1.866621007194245e-4)+t7.*t23.*1.0./t54.^19.*6.454925057900768e-29+t2.*t30.^(1.1e+1./2.5e+1).*t47.*1.408065768852544e-7;
et5 = t3.*t47.*t71.^8.*1.139466607056987e-11+t2.*t23.*1.0./t30.^(1.03e+2./1.0e+2).*1.13884790987354e-9+rho.*t8.*t127.*2.528445291510791e-1;
et6 = rho.*t10.*t127.*(-2.634424805992931e+4)+rho.*t46.*t124.*9.466435107913669e-4-t3.*t8.*t117.*9.315164430883049e-7;
et7 = t2.*t42.*t115.*(-1.725223202732778e-10)+t2.*t45.*t115.*4.258836706174629e-9+t3.*t42.*t128.*2.383457690483743e-11-t3.*t45.*t128.*4.8486339303555e-12;
et8 = t3.*t66.*t117.*(-3.165408600952511e-11)-rho.*t9.*t105.*t127.*9.300886004822446e+1+rho.*t43.*t96.*t124.*9.333105035971223e-4+t2.*t44.*t80.*t115.*1.380178562186222e-10;
et9 = t3.*t44.*t102.*t128.*(-1.906766152386994e-11)+rho.*t10.*t105.^2.*t127.*5.702218194789895e+3-rho.*t46.*t96.^2.*t124.*3.333251798561151e-4;
et10 = t3.*t8.*t66.^2.*t117.*5.821977769301905e-9-t2.*t45.*t80.^2.*t115.*1.971683660266032e-11+t3.*t45.*t102.^2.*t128.*2.723951646267135e-12;
et11 = t65.*9.65567e-1+t137+t144-rho.*t61.*2.529528057553957e-4-t2.*t8.*1.165829442609941e-5-t23.*t76.*1.3610524;
et12 = t47.*t64.*1.393711-t45.*t115.*6.857082e-4+t86.*t153+t91.*t158+t99.*t159+rho.*t23.*t76.*6.527829256594724e-4+rho.*t47.*t62.*8.887890647482015e-4;
et13 = rho.*t47.*t63.*(-1.741015827338129e-3)+rho.*t8.*t117.*6.074267353956834e-1-rho.*t10.*t127.*1.52363270164786e+4+rho.*t46.*t124.*6.799833669064748e-4;
et14 = rho.*t45.*t128.*2.841991366906475e-4+t5.*t23.*t57.*8.979523707146454e-19-t6.*t23.*t57.*7.177876664385654e-23;
et15 = t3.*t47.*t62.*(-1.192623542075196e-10)-t2.*t47.*t64.*4.007473158164116e-7+t3.*t47.*t63.*6.674816798218516e-11+t5.*t47.*t62.*1.95958101691341e-18;
et16 = t4.*t47.*t64.*9.218462716247988e-15-t3.*t8.*t117.*6.800070034544626e-8+t2.*t45.*t115.*6.388255059261943e-10;
et17 = t3.*t45.*t128.*(-5.747537973623655e-12)-t10.*t91.*t127.*4.755649974454772e+7+t46.*t77.*t124.*2.779932+rho.*t45.*t68.*t115.*3.288768345323741e-7;
et18 = t2.*t8.*t86.*t117.*(-1.456658837879337e-4)-t2.*t45.*t99.*t128.*6.815327018960372e-8-rho.*t46.*t77.^2.*t124.*3.333251798561151e-4-t2.*t45.*t68.^2.*t115.*1.971683660266032e-11;
et19 = t3.*2.533418566459739e-12-t47.*t59.*2.75881368-t2.*t117.*1.979963079895795e-7-t9.*t127.*1.93923473200548e+5;
et20 = t43.*t124.*1.9459524+t66.*t145+t80.*t154+t96.*t156+t102.*t151+t105.*t149-rho.*t71.^2.*2.176577889688249e-4+t2.*1.0./t30.^(3.1e+1./5.0e+1).*1.152542760036575e-8+1.0./t30.^(1.7e+1./2.5e+1).*4.9502656e-1;
et21 = 1.0./t30.^(7.1e+1./1.0e+3).*(-2.188015173)+rho.*t23.*t71.*3.165997189448441e-4-rho.*t47.*t60.*8.155047577937649e-4+rho.*t44.*t115.*5.755344604316547e-7;
et22 = t6.*t23.*t54.*(-3.768385248802469e-23)+t7.*t23.*t54.*1.290985011580154e-27-t2.*t23.*t71.*3.796159699578467e-8;
et23 = t2.*t47.*t58.*(-1.875622007142488e-7)+t2.*t47.*t59.*3.173074409537118e-7+t4.*t47.*t58.*7.190878499665448e-15+t3.*t47.*t60.*4.689800722264001e-11;
et24 = t2.*t44.*t128.*(-1.192682228318065e-7)+t3.*t86.*t117.*1.582704300476255e-11-t46.*t96.*t124.*1.389966+rho.*t9.*t91.*t127.*4.650443002411223e+1;
et25 = rho.*t45.*t80.*t115.*(-1.644384172661871e-7)-rho.*t43.*t77.*t124.*4.666552517985612e-4-t2.*t44.*t68.*t115.*6.900892810931111e-11+t3.*t44.*t99.*t128.*9.533830761934972e-12;
et26 = rho.*t10.*t91.*t105.*t127.*(-5.702218194789895e+3)-t3.*t8.*t66.*t86.*t117.*5.821977769301905e-9-t3.*t45.*t99.*t102.*t128.*2.723951646267135e-12;
cp = t9.*(et1+et2+et3+et4+et5+et6+et7+et8+et9+et10).*1.12506132549482e+6+((t11.*t160-rho.*t8.*(et19+et20+et21+et22+et23+et24+et25+et26).*8.821342925659472e-2+1.0).^2.*8.314472)./((rho.*t160)./2.085e+3-(t2.*(et11+et12+et13+et14+et15+et16+et17+et18))./1.73889e+7+1.0);
end

== matlab function base_lib/F0021_R1234yf/F0021_cv.m ==
  data: T input; cv output; rho input
function cv = F0021_cv(T,rho)
%R1234yf_cv
%    CV = R1234yf_cv(T,RHO)

%    This function was generated by the Symbolic Math Toolbox version 9.3.
%    16-Oct-2023 15:47:50

t2 = rho.^2;
t3 = rho.^3;
t4 = 1.0./T;
t7 = rho./4.17e+3;
t5 = t4.^2;
t6 = t4.^3;
t8 = t4.*7.18e+2;
t9 = t4.*8.77e+2;
t10 = t4.*1.755e+3;
t11 = t4.*4.465e+3;
t12 = -t7;
t17 = t4.*5.8856e+4;
t23 = t4.*3.6785e+2;
t24 = t4.*7.94556e+4;
t25 = t2./1.73889e+7;
t30 = t4.*1.044694e+3;
t31 = t7-4.1e+1./2.5e+1;
t38 = t4.*6.54773e+2;
t39 = t4.*1.699467e+3;
t40 = t7-9.1e+1./1.0e+2;
t41 = t7-8.9e+1./1.25e+2;
t42 = t7-3.59e+2./5.0e+2;
t46 = t7-6.77e+2./1.0e+3;
t13 = -t8;
t14 = -t9;
t15 = -t10;
t16 = -t11;
t18 = exp(t12);
t32 = -t25;
t33 = t23.^(3.0./2.0);
t34 = t23.^(5.0./2.0);
t35 = t23.^(7.0./2.0);
t36 = t23.^(7.0./5.0);
t43 = t23-6.0./5.0;
t44 = t31.^2;
t45 = t17-2.048e+2;
t47 = t23-3.2e+1./2.5e+1;
t48 = t23-2.3e+1./5.0e+1;
t49 = t40.^2;
t50 = t41.^2;
t51 = t42.^2;
t53 = t23-6.7e+1./1.0e+2;
t54 = t23-1.13e+2./1.0e+2;
t55 = t24-2.592e+2;
t56 = t46.^2;
t68 = t30-3.2092;
t73 = t38-8.188e-1;
t76 = t39-3.0954;
t19 = exp(t13);
t20 = exp(t14);
t21 = exp(t15);
t22 = exp(t16);
t37 = exp(t32);
t52 = t43.^2;
t57 = t47.^2;
t58 = t48.^2;
t60 = t53.^2;
t61 = t54.^2;
t62 = t44.*(8.1e+1./5.0);
t66 = t50.*(5.1e+1./5.0e+1);
t70 = t51.*(1.46e+2./2.5e+1);
t71 = t49.*(1.67e+2./1.25e+2);
t77 = t56.*(2.11e+2./2.0e+2);
t26 = t19-1.0;
t27 = t20-1.0;
t28 = t21-1.0;
t29 = t22-1.0;
t59 = t52.*1.08e+2;
t64 = -t62;
t65 = t57.*8.0e+1;
t69 = -t66;
t72 = -t70;
t74 = -t71;
t75 = t58.*(8.9e+1./1.0e+2);
t79 = t61.*(7.1e+1./5.0e+1);
t80 = -t77;
t82 = t60.*(2.31e+2./1.0e+2);
t63 = -t59;
t67 = -t65;
t78 = -t75;
t81 = -t79;
t83 = -t82;
t84 = t63+t64;
t86 = t67+t72;
t88 = t69+t81;
t90 = t74+t83;
t91 = t78+t80;
t85 = exp(t84);
t87 = exp(t86);
t89 = exp(t88);
t92 = exp(t90);
t93 = exp(t91);
et1 = 1.0./t26.^2.*exp(t4.*-1.436e+3).*2.876052391546904e+1+1.0./t27.^2.*exp(t4.*-1.754e+3).*8.736380352244283+1.0./t28.^2.*exp(t4.*-3.51e+3).*1.696916093943165e+2+1.0./t29.^2.*exp(t4.*-8.93e+3).*2.990869359808914e+2+rho.*1.0./t23.^(4.2e+1./2.5e+1).*8.072375558752998e-5;
et2 = rho.*1.0./t23.^1.071.*(-3.72539753676259e-5)-(t19.*2.876052391546904e+1)./t26-(t20.*8.736380352244283)./t27-(t21.*1.696916093943165e+2)./t28-(t22.*2.990869359808914e+2)./t29;
et3 = t2.*1.0./t23.^(5.3e+1./5.0e+1).*(-1.565883373876438e-9)+t3.*1.0./t23.^(8.1e+1./5.0e+1).*5.712042455816759e-13+3.653734124219459e-5./t5+rho.*t23.^(7.0./2.5e+1).*t37.*8.468300984172661e-4;
et4 = rho.*1.0./t23.^(3.0./5.0).*t89.*(-1.866621007194245e-4)+t3.*1.0./t23.^(6.0./2.5e+1).*t37.*1.139466607056987e-11+t2.*t23.^(1.1e+1./2.5e+1).*t37.*1.408065768852544e-7;
et5 = t2.*t18.*1.0./t23.^(1.03e+2./1.0e+2).*1.13884790987354e-9+rho.^7.*t18.*1.0./t23.^(1.9e+1./2.0e+1).*6.454925057900768e-29+rho.*t4.*t92.*2.528445291510791e-1;
et6 = rho.*t6.*t92.*(-2.634424805992931e+4)+rho.*t36.*t89.*9.466435107913669e-4-t3.*t4.*t87.*9.315164430883049e-7;
et7 = t2.*t33.*t85.*(-1.725223202732778e-10)+t2.*t35.*t85.*4.258836706174629e-9+t3.*t33.*t93.*2.383457690483743e-11-t3.*t35.*t93.*4.8486339303555e-12;
et8 = t3.*t45.*t87.*(-3.165408600952511e-11)-rho.*t5.*t76.*t92.*9.300886004822446e+1+t2.*t34.*t55.*t85.*1.380178562186222e-10-t3.*t34.*t73.*t93.*1.906766152386994e-11;
et9 = rho.*t6.*t76.^2.*t92.*5.702218194789895e+3+rho.*t23.^(2.0./5.0).*t68.*t89.*9.333105035971223e-4-rho.*t36.*t68.^2.*t89.*3.333251798561151e-4;
et10 = t3.*t4.*t45.^2.*t87.*5.821977769301905e-9-t2.*t35.*t55.^2.*t85.*1.971683660266032e-11+t3.*t35.*t73.^2.*t93.*2.723951646267135e-12;
cv = t5.*(et1+et2+et3+et4+et5+et6+et7+et8+et9+et10).*1.12506132549482e+6;
end

== matlab function base_lib/F0021_R1234yf/F0021_dliqsat.m ==
  data: T input; dliq output
function dliq = F0021_dliqsat(T)
% correlation from Martin (1959)


% critical Temp & density
Tc   =     367.85; % [K]
rhoc =     4170.0; % [mol/m3]

T = min(T, Tc);
T = max(T, 0);

% coefficients
x = [   1.768478200876913;
        0.905584244505430;
       -0.353914488877852;
        0.447866446078125 ];

% saturated liquid dfensity
Tr   = T ./ Tc;
A    = [ (1-Tr).^(1/3), (1-Tr).^(2/3), (1-Tr), (1-Tr).^(4/3) ];
dliq = rhoc .* ( 1 + A * x );


end

== matlab function base_lib/F0021_R1234yf/F0021_dpdrho.m ==
  data: T input; dp_drho output; rho input
function dp_drho = R1234yf_dpdrho(T,rho)
%R1234yf_dpdrho
%    DP_DRHO = R1234yf_dpdrho(T,RHO)

%    This function was generated by the Symbolic Math Toolbox version 9.3.
%    27-Oct-2023 18:05:02

t2 = rho.^2;
t3 = rho.^3;
t5 = rho.^5;
t7 = rho.^7;
t8 = 1.0./T;
t10 = rho./4.17e+3;
t11 = rho.*7.769784172661871e-3;
t14 = rho.*4.892086330935252e-4;
t15 = rho.*2.800959232613909e-3;
t17 = rho.*6.407673860911271e-4;
t18 = rho.*5.059952038369305e-4;
t4 = t2.^2;
t6 = t2.^3;
t9 = t8.^3;
t12 = -t10;
t16 = t8.*3.6785e+2;
t19 = t2./1.73889e+7;
t20 = t10-4.1e+1./2.5e+1;
t25 = t10-9.1e+1./1.0e+2;
t26 = t10-8.9e+1./1.25e+2;
t27 = t10-3.59e+2./5.0e+2;
t36 = t10-6.77e+2./1.0e+3;
t37 = t11-5.3136e+1;
t45 = t14-1.45248;
t52 = t15-8.38624;
t57 = t17-2.43152;
t64 = t18-1.42847;
t13 = exp(t12);
t21 = -t19;
t22 = t16.^(7.0./2.0);
t23 = t16.^(7.0./5.0);
t28 = t16-6.0./5.0;
t29 = t20.^2;
t30 = t16.^(2.1e+1./2.0e+1);
t31 = t16.^(1.9e+1./5.0e+1);
t32 = t16.^(4.4e+1./2.5e+1);
t34 = t16.^(6.1e+1./2.5e+1);
t35 = t16.^(4.7e+1./5.0e+1);
t38 = t16-3.2e+1./2.5e+1;
t39 = t16-2.3e+1./5.0e+1;
t40 = t25.^2;
t41 = t26.^2;
t42 = t27.^2;
t44 = t16.^(9.7e+1./1.0e+2);
t46 = t16-6.7e+1./1.0e+2;
t47 = t16-1.13e+2./1.0e+2;
t48 = t36.^2;
t24 = exp(t21);
t33 = t31.^6;
t43 = t28.^2;
t49 = t38.^2;
t50 = t39.^2;
t53 = t46.^2;
t54 = t47.^2;
t55 = t29.*(8.1e+1./5.0);
t60 = t41.*(5.1e+1./5.0e+1);
t63 = t42.*(1.46e+2./2.5e+1);
t65 = t40.*(1.67e+2./1.25e+2);
t69 = t48.*(2.11e+2./2.0e+2);
t86 = t2.*t13.*t44.*3.913566700596357e-8;
t88 = t7.*t13.*t30.*1.229509534838242e-27;
t51 = t43.*1.08e+2;
t58 = -t55;
t59 = t49.*8.0e+1;
t62 = -t60;
t66 = -t63;
t67 = -t65;
t68 = t50.*(8.9e+1./1.0e+2);
t71 = t54.*(7.1e+1./5.0e+1);
t72 = -t69;
t74 = t53.*(2.31e+2./1.0e+2);
t87 = -t86;
t56 = -t51;
t61 = -t59;
t70 = -t68;
t73 = -t71;
t75 = -t74;
t76 = t56+t58;
t78 = t61+t66;
t80 = t62+t73;
t82 = t67+t75;
t83 = t70+t72;
t77 = exp(t76);
t79 = exp(t78);
t81 = exp(t80);
t84 = exp(t82);
t85 = exp(t83);
et1 = t87+t88-rho.*t35.*2.315508393285372e-4+t3.*t8.*9.319180196722149e-10+t2.*t31.*3.033007263254145e-8-t24.*t33.*1.210006;
et2 = t9.*t84.*(-2.377824987227386e+7)+t23.*t81.*1.389966+t16.^(8.0./2.5e+1).*1.546958-t16.^(9.29e+2./1.0e+3).*2.355237;
et3 = rho.*t13.*t44.*3.263914628297362e-4-rho.*t24.*t34.*3.342232613908873e-4+rho.*t22.*t77.*1.644384172661871e-7-t6.*t13.*t30.*3.588938332192827e-23;
et4 = t2.*t24.*t32.*(-1.06569432224005e-7)+t2.*t24.*t33.*1.391699302428561e-7+t4.*t24.*t32.*4.085726420264459e-15+t3.*t24.*t34.*1.922049476337705e-11;
et5 = t2.*t8.*t79.*(-7.283294189396684e-5)-t2.*t22.*t85.*3.407663509480186e-8-rho.*t23.*t45.*t81.*3.333251798561151e-4+rho.*t9.*t57.*t84.*5.702218194789895e+3;
et6 = t2.*t22.*t37.*t77.*(-1.971683660266032e-11)+t3.*t8.*t52.*t79.*5.821977769301905e-9+t3.*t22.*t64.*t85.*2.723951646267135e-12;
et7 = t35.*9.65567e-1+t87+t88-rho.*t31.*2.529528057553957e-4-t2.*t8.*1.165829442609941e-5-t13.*t44.*1.3610524;
et8 = t24.*t34.*1.393711-t22.*t77.*6.857082e-4+rho.*t24.*t32.*8.887890647482015e-4+rho.*t13.*t44.*6.527829256594724e-4-rho.*t24.*t33.*1.741015827338129e-3;
et9 = rho.*t8.*t79.*6.074267353956834e-1-rho.*t9.*t84.*1.52363270164786e+4+rho.*t23.*t81.*6.799833669064748e-4+rho.*t22.*t85.*2.841991366906475e-4;
et10 = t5.*t13.*t30.*8.979523707146454e-19-t6.*t13.*t30.*7.177876664385654e-23-t3.*t24.*t32.*1.192623542075196e-10;
et11 = t2.*t24.*t34.*(-4.007473158164116e-7)+t3.*t24.*t33.*6.674816798218516e-11+t5.*t24.*t32.*1.95958101691341e-18+t4.*t24.*t34.*9.218462716247988e-15;
et12 = t3.*t8.*t79.*(-6.800070034544626e-8)+t2.*t22.*t77.*6.388255059261943e-10-t3.*t22.*t85.*5.747537973623655e-12+t23.*t45.*t81.*2.779932;
et13 = t9.*t57.*t84.*(-4.755649974454772e+7)+rho.*t22.*t37.*t77.*3.288768345323741e-7-t2.*t8.*t52.*t79.*1.456658837879337e-4-t2.*t22.*t64.*t85.*6.815327018960372e-8;
et14 = rho.*t23.*t45.^2.*t81.*(-3.333251798561151e-4)+rho.*t9.*t57.^2.*t84.*5.702218194789895e+3-t2.*t22.*t37.^2.*t77.*1.971683660266032e-11;
et15 = t3.*t8.*t52.^2.*t79.*5.821977769301905e-9+t3.*t22.*t64.^2.*t85.*2.723951646267135e-12;
dp_drho = T.*((rho.*(et1+et2+et3+et4+et5+et6))./2.085e+3-(t2.*(et7+et8+et9+et10+et11+et12+et13+et14+et15))./1.73889e+7+1.0).*8.314472;
end
